simulink model "ex1_model"  (R2015b)
settings: Solver=FixedStepAuto  StartTime=0.0  StopTime=300  FixedStep=0.1  RelTol=1e-3
values from neighbouring files (symbols this model uses):
  a = A(i)    [ex1_script.m]
  b = B(j)    [ex1_script.m]
settings Model: Creator=Tomáš  LastModifiedBy=Tomáš

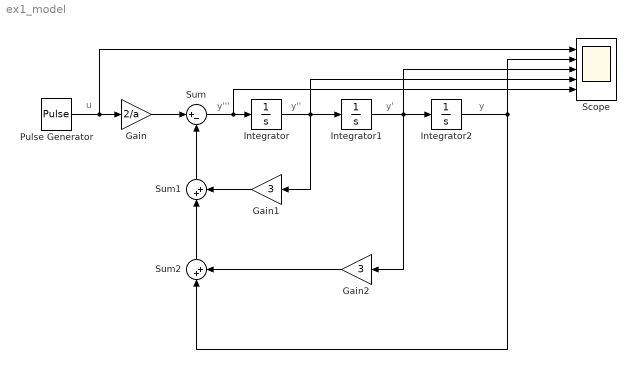
== system ex1_model ==
  note: y
  note: y'
  note: y''
  note: y'''
  note: u
  Gain : Gain  Gain=2/a
  Gain1 : Gain  Gain=3
  Gain2 : Gain  Gain=3
  Integrator : Integrator  InitialCondition=b
  Integrator1 : Integrator  InitialCondition=2*b
  Integrator2 : Integrator  InitialCondition=3*b
  Pulse Generator : DiscretePulseGenerator  PulseType=Time based  Period=100  PulseWidth=50
  Scope : Scope  NumInputPorts=5
  Sum : Sum  Inputs=|+-
  Sum1 : Sum  Inputs=|++
  Sum2 : Sum  Inputs=|++
  wires:
  Integrator1/1 -> Scope/3, Gain2/1, Integrator2/1
  Integrator/1 -> Scope/4, Gain1/1, Integrator1/1
  Sum/1 -> Integrator/1, Scope/5
  Pulse Generator/1 -> Gain/1, Scope/1
  Gain/1 -> Sum/1
  Gain1/1 -> Sum1/2
  Sum1/1 -> Sum/2
  Sum2/1 -> Sum1/1
  Gain2/1 -> Sum2/2
  Integrator2/1 -> Sum2/1, Scope/2
